simulink model "Simulation_Project_2015297"  (R2016a)
settings: Solver=VariableStepAuto  StartTime=0.0  StopTime=10.0  MaxStep=0.05  RelTol=1e-3
settings Model: Creator=hp  LastModifiedBy=hp

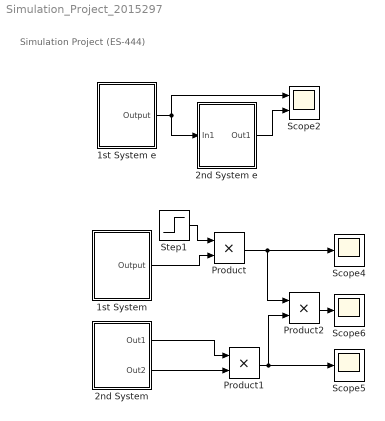
== system Simulation_Project_2015297 ==
  note: Simulation Project (ES-444)
  1st System : Subsystem  mask{omega_initial=0, theta=40, m=1, l=1, d=1.5, g=9.8}
      mask prompts: omega_initial "Initial_Angular _Velocity(Omega)"; theta "Initial_Angular_Displacement(Degree)"; m "Mass"; l "Length of String(l)"; d "Damping Coefficient(d)"; g "Gravity(g)"
  1st System e : Subsystem  mask{omega_initial=0, theta=40, m=1, l=1, d=1.5, g=9.8}
      mask prompts: omega_initial "Initial_Angular _Velocity(Omega)"; theta "Initial_Angular_Displacement(Degree)"; m "Mass"; l "Length of String(l)"; d "Damping Coefficient(d)"; g "Gravity(g)"
  2nd System : Subsystem  mask{theta=90}
      mask prompts: theta "Initial_Angular_Displacement(Degree)"
  2nd System e : Subsystem  mask{theta=0.9, l=1, d=2, m=1}
      mask prompts: l "Length"; d "Damping Coefficient"; m "Mass"
  Product : Product
  Product1 : Product
  Product2 : Product
  Scope2 : Scope  NumInputPorts=2
  Scope4 : Scope
  Scope5 : Scope
  Scope6 : Scope
  Step1 : Step  SampleTime=0
  wires:
  1st System e/1(Output) -> 2nd System e/1(In1), Scope2/1
  2nd System e/1(Out1) -> Scope2/2
  1st System/1(Output) -> Product/2
  Step1/1 -> Product/1
  Product/1 -> Product2/1, Scope4/1
  Product1/1 -> Scope5/1, Product2/2
  Product2/1 -> Scope6/1
  2nd System/1(Out1) -> Product1/1
  2nd System/2(Out2) -> Product1/2

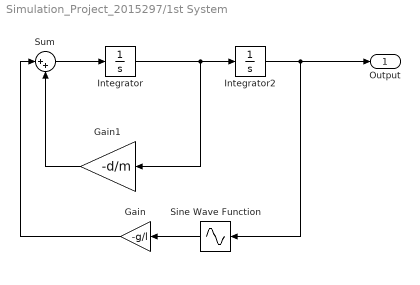
== system Simulation_Project_2015297/1st System ==
  Gain : Gain  Gain=-g/l
  Gain1 : Gain  Gain=-d/m
  Integrator : Integrator  InitialCondition=omega_initial
  Integrator2 : Integrator  InitialCondition=theta*pi/180
  Sine Wave Function : Sin  TimeSource=Use external signal  SampleTime=0
  Sum : Sum  Inputs=|++
  Output : Outport
  wires:
  Sum/1 -> Integrator/1
  Integrator/1 -> Gain1/1, Integrator2/1
  Gain/1 -> Sum/1
  Integrator2/1 -> Output/1, Sine Wave Function/1
  Sine Wave Function/1 -> Gain/1
  Gain1/1 -> Sum/2

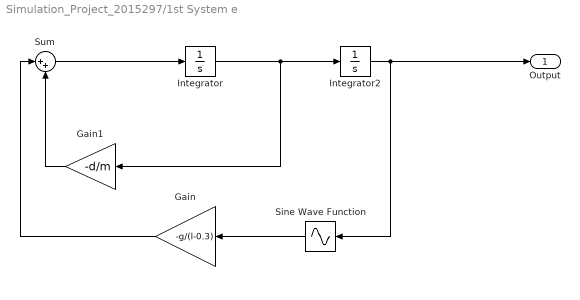
== system Simulation_Project_2015297/1st System e ==
  Gain : Gain  Gain=-g/(l-0.3)
  Gain1 : Gain  Gain=-d/m
  Integrator : Integrator  InitialCondition=omega_initial
  Integrator2 : Integrator  InitialCondition=theta*pi/180
  Sine Wave Function : Sin  TimeSource=Use external signal  SampleTime=0
  Sum : Sum  Inputs=|++
  Output : Outport
  wires:
  Integrator/1 -> Gain1/1, Integrator2/1
  Sum/1 -> Integrator/1
  Gain/1 -> Sum/1
  Integrator2/1 -> Output/1, Sine Wave Function/1
  Sine Wave Function/1 -> Gain/1
  Gain1/1 -> Sum/2

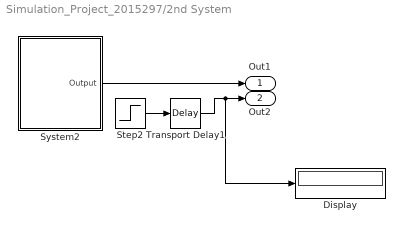
== system Simulation_Project_2015297/2nd System ==
  Display : Display
  Step2 : Step  SampleTime=0
  System2 : Subsystem  mask{omega_initial=0, theta=30, m=1, l=1, d=1.5, g=9.8}
      mask prompts: omega_initial "Initial_Angular _Velocity(Omega)"; theta "Initial_Angular_Displacement(Degree)"; m "Mass"; l "Length of String(l)"; d "Damping Coefficient(d)"; g "Gravity(g)"
  Transport Delay1 : TransportDelay  DelayTime=theta*(3.14)/180
  Out1 : Outport
  Out2 : Outport  Port=2
  wires:
  System2/1(Output) -> Out1/1
  Transport Delay1/1 -> Display/1, Out2/1
  Step2/1 -> Transport Delay1/1

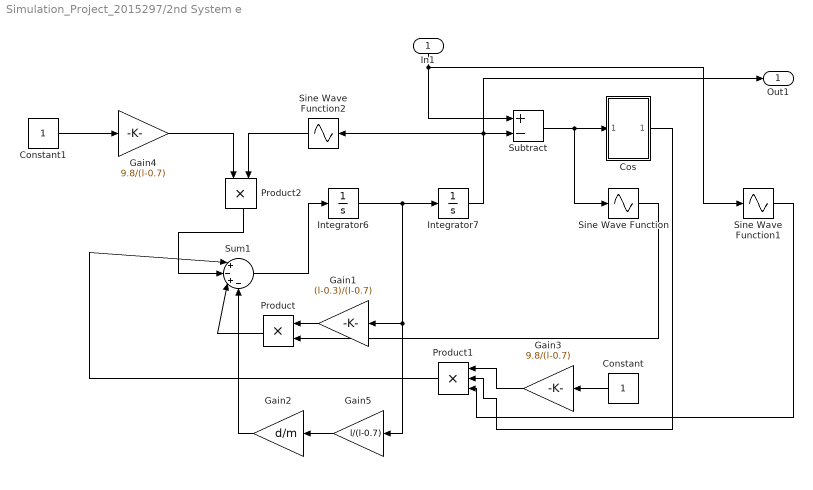
== system Simulation_Project_2015297/2nd System e ==
  In1 : Inport
  Constant : Constant
  Constant1 : Constant
  Cos : Subsystem
  Gain1 : Gain  Gain=(l-0.3)/(l-0.7)
  Gain2 : Gain  Gain=d/m
  Gain3 : Gain  Gain=9.8/(l-0.7)
  Gain4 : Gain  Gain=9.8/(l-0.7)
  Gain5 : Gain  Gain=l/(l-0.7)
  Integrator6 : Integrator  InitialCondition=1
  Integrator7 : Integrator  InitialCondition=theta
  Product : Product
  Product1 : Product  Inputs=3
  Product2 : Product
  Sine Wave Function : Sin  TimeSource=Use external signal  SampleTime=0
  Sine Wave Function1 : Sin  TimeSource=Use external signal  SampleTime=0
  Sine Wave Function2 : Sin  TimeSource=Use external signal  SampleTime=0
  Subtract : Sum  Inputs=+-
  Sum1 : Sum  Inputs=|+-+-
  Out1 : Outport
  wires:
  Integrator7/1 -> Out1/1, Sine Wave Function2/1, Subtract/2
  Integrator6/1 -> Integrator7/1, Gain5/1, Gain1/1
  Product/1 -> Sum1/3
  Sum1/1 -> Integrator6/1
  Gain4/1 -> Product2/1
  Product1/1 -> Sum1/1
  Product2/1 -> Sum1/2
  Gain1/1 -> Product/1
  Cos/1(Out1) -> Product1/2
  Constant/1 -> Gain3/1
  Sine Wave Function1/1 -> Product1/3
  Gain3/1 -> Product1/1
  Sine Wave Function2/1 -> Product2/2
  Constant1/1 -> Gain4/1
  Sine Wave Function/1 -> Product/2
  Subtract/1 -> Sine Wave Function/1, Cos/1(In1)
  In1/1 -> Sine Wave Function1/1, Subtract/1
  Gain5/1 -> Gain2/1
  Gain2/1 -> Sum1/4

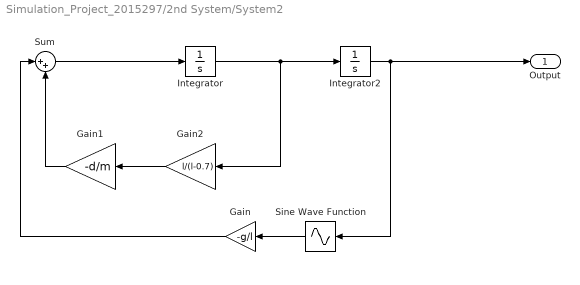
== system Simulation_Project_2015297/2nd System/System2 ==
  Gain : Gain  Gain=-g/l
  Gain1 : Gain  Gain=-d/m
  Gain2 : Gain  Gain=l/(l-0.7)
  Integrator : Integrator  InitialCondition=omega_initial
  Integrator2 : Integrator  InitialCondition=theta*pi/180
  Sine Wave Function : Sin  TimeSource=Use external signal  SampleTime=0
  Sum : Sum  Inputs=|++
  Output : Outport
  wires:
  Gain1/1 -> Sum/2
  Sine Wave Function/1 -> Gain/1
  Integrator2/1 -> Sine Wave Function/1, Output/1
  Gain/1 -> Sum/1
  Integrator/1 -> Integrator2/1, Gain2/1
  Sum/1 -> Integrator/1
  Gain2/1 -> Gain1/1

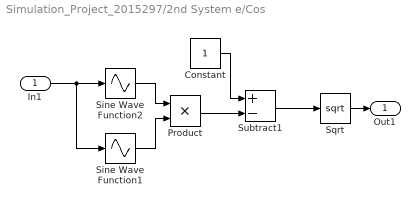
== system Simulation_Project_2015297/2nd System e/Cos ==
  In1 : Inport
  Constant : Constant
  Product : Product
  Sine Wave Function1 : Sin  TimeSource=Use external signal  SampleTime=0
  Sine Wave Function2 : Sin  TimeSource=Use external signal  SampleTime=0
  Sqrt : Sqrt  SaturateOnIntegerOverflow=on
  Subtract1 : Sum  Inputs=+-
  Out1 : Outport
  wires:
  Subtract1/1 -> Sqrt/1
  Product/1 -> Subtract1/2
  Sine Wave Function1/1 -> Product/2
  In1/1 -> Sine Wave Function1/1, Sine Wave Function2/1
  Sqrt/1 -> Out1/1
  Constant/1 -> Subtract1/1
  Sine Wave Function2/1 -> Product/1
